simulink model "quadcopter_model"  (R2020b)
settings: Solver=VariableStepAuto  StartTime=0.0  StopTime=40  MaxStep=1e-3  RelTol=1e-3
values from neighbouring files (symbols this model uses):
  g = 9.81    [model_parameters.m]    (also in state_fcn.m = [0; 0; 9.81]; state_fcn1.m = [0; 0; 9.81])
  J = diag([Jxx, Jyy, Jzz])    [model_parameters.m]    (also in state_fcn1.m)
  JR = 1e-5    (= 1e-05)    [model_parameters.m]    (also in state_fcn1.m)
  Kv = 980    [model_parameters.m]
  m = 0.6    [model_parameters.m]    (also in state_fcn1.m)
  Omega_b = 0    [model_parameters.m]
  S = [cT cT cT cT ... (first row only)    [model_parameters.m]    (also in state_fcn1.m = [       cT              cT              cT              cT)
  Tm = 0.02    [model_parameters.m]
  Ts = 0.1    [linear_mpc.m]
  Ub = 12    [model_parameters.m]
libraries: simulink x5, eeStairGenerator x4, sharedutil x3, mpclib x1, robotcorelib x1
settings Model: Creator=Bojan  LastModifiedBy=Bojan Derajic

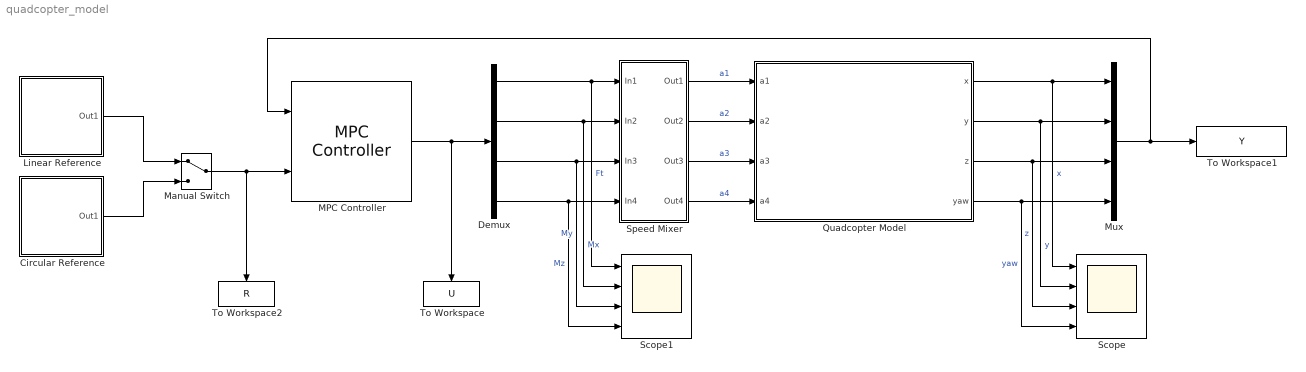
== system quadcopter_model ==
  Circular Reference : Subsystem
  Demux : Demux
  Linear Reference : Subsystem
  MPC Controller : mpclib/MPC Controller  SCDEnableBlockLinearizationSpecification=on  mpcobj=MPC_lin  is_multiple=0  enable_value=0  return_u0=off  updateMPCinCallerWorkspace=on  md_inport=off  mv_inport=off  uref_inport=off  return_cost=off  return_mvseq=off  return_qpstatus=off  return_xseq=off  return_state=off  return_ovseq=off  state_inport=off  umin_inport=off  umax_inport=off  ymin_inport=off  ymax_inport=off  cc_inport=off  ywt_inport=off  uwt_inport=off  duwt_inport=off  rhoeps_inport=off  pm_inport=off  MaximumP=10  HorizonChoice=FixedHorizon  n_ts=0.1  n_p=60  n_mv=4  n_md=0  n_ud=0  n_mo=4  n_uo=0  BlockDataType=double  SampleTimeInherited=off  switch_inport=off
  Manual Switch : ManualSwitch
  Mux : Mux
  Quadcopter Model : Subsystem
      mask Display: image('C:\Users\Bojan Derajic\OneDrive\Master studije - Predmeti BG\Robotski sistemi (13M051RS)\Quadcopter model\icons\quadcopter.jpg'); % Use "Edit Image" on toolstrip to change.
  Scope : Scope  NumInputPorts=4
  Scope1 : Scope  NumInputPorts=4
  Speed Mixer : Subsystem
  To Workspace : ToWorkspace  VariableName=U  SaveFormat=Structure With Time  SampleTime=-1
  To Workspace1 : ToWorkspace  VariableName=Y  SaveFormat=Structure With Time  SampleTime=-1
  To Workspace2 : ToWorkspace  VariableName=R  SaveFormat=Structure With Time  SampleTime=-1
  wires:
  Speed Mixer/4(Out4) -> Quadcopter Model/4(a4)  "a4"
  Speed Mixer/3(Out3) -> Quadcopter Model/3(a3)  "a3"
  Speed Mixer/2(Out2) -> Quadcopter Model/2(a2)  "a2"
  Speed Mixer/1(Out1) -> Quadcopter Model/1(a1)  "a1"
  Quadcopter Model/1(x) -> Scope/1, Mux/1  "x"
  Quadcopter Model/2(y) -> Mux/2, Scope/2  "y"
  Quadcopter Model/3(z) -> Mux/3, Scope/3  "z"
  Quadcopter Model/4(yaw) -> Mux/4, Scope/4  "yaw"
  Mux/1 -> To Workspace1/1, MPC Controller/1
  Demux/1 -> Scope1/1, Speed Mixer/1(In1)  "Ft"
  Demux/2 -> Scope1/2, Speed Mixer/2(In2)  "Mx"
  Demux/3 -> Scope1/3, Speed Mixer/3(In3)  "My"
  Demux/4 -> Scope1/4, Speed Mixer/4(In4)  "Mz"
  MPC Controller/1 -> To Workspace/1, Demux/1
  Manual Switch/1 -> MPC Controller/2, To Workspace2/1
  Linear Reference/1(Out1) -> Manual Switch/1
  Circular Reference/1(Out1) -> Manual Switch/2

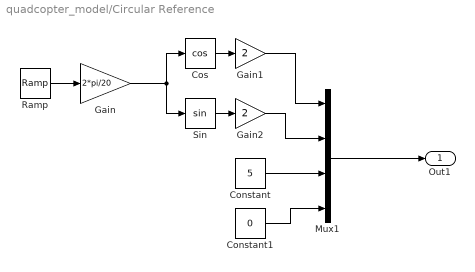
== system quadcopter_model/Circular Reference ==
  Constant : Constant  Value=5
  Constant1 : Constant  Value=0
  Cos : Trigonometry  Operator=cos
  Gain : Gain  Gain=2*pi/20
  Gain1 : Gain  Gain=2
  Gain2 : Gain  Gain=2
  Mux1 : Mux
  Ramp : simulink/Sources/Ramp  slope=1  start=5  InitialOutput=0
  Sin : Trigonometry
  Out1 : Outport
  wires:
  Gain1/1 -> Mux1/1
  Gain2/1 -> Mux1/2
  Cos/1 -> Gain1/1
  Sin/1 -> Gain2/1
  Ramp/1 -> Gain/1
  Mux1/1 -> Out1/1
  Constant/1 -> Mux1/3
  Gain/1 -> Sin/1, Cos/1
  Constant1/1 -> Mux1/4

== system quadcopter_model/Linear Reference ==
  Mux1 : Mux
  Stair Generator : eeStairGenerator/Stair Generator  LabelModeActiveChoice=Discrete  TimeInput=[5, 15]  AmplitudeInput=[-2, 3]  SampleTime=Ts  RepeatPattern=off  OutDataTypeStr=double
      settings: SourceProductBaseCode=PS
  Stair Generator1 : eeStairGenerator/Stair Generator  LabelModeActiveChoice=Discrete  TimeInput=[0, 24]  AmplitudeInput=[5, 0]  SampleTime=Ts  RepeatPattern=off  OutDataTypeStr=double
      settings: SourceProductBaseCode=PS
  Stair Generator2 : eeStairGenerator/Stair Generator  LabelModeActiveChoice=Discrete  TimeInput=[20]  AmplitudeInput=[0.1]  SampleTime=Ts  RepeatPattern=off  OutDataTypeStr=double
      settings: SourceProductBaseCode=PS
  Stair Generator3 : eeStairGenerator/Stair Generator  LabelModeActiveChoice=Discrete  TimeInput=[10]  AmplitudeInput=[5]  SampleTime=Ts  RepeatPattern=off  OutDataTypeStr=double
      settings: SourceProductBaseCode=PS
  Out1 : Outport
  wires:
  Stair Generator1/1 -> Mux1/3
  Stair Generator/1 -> Mux1/2
  Stair Generator2/1 -> Mux1/4
  Mux1/1 -> Out1/1
  Stair Generator3/1 -> Mux1/1

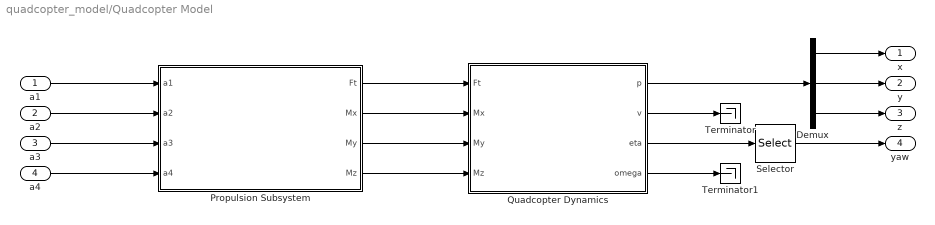
== system quadcopter_model/Quadcopter Model ==
  a1 : Inport
  a2 : Inport  Port=2
  a3 : Inport  Port=3
  a4 : Inport  Port=4
  Demux : Demux  Outputs=3
  Propulsion Subsystem : Subsystem
  Quadcopter Dynamics : Subsystem
  Selector : Selector  InputPortWidth=3  IndexOptions=Index vector (dialog)  Indices=[3]  OutputSizes=1
  Terminator : Terminator
  Terminator1 : Terminator
  x : Outport
  y : Outport  Port=2
  z : Outport  Port=3
  yaw : Outport  Port=4
  wires:
  Propulsion Subsystem/1(Ft) -> Quadcopter Dynamics/1(Ft)
  a4/1 -> Propulsion Subsystem/4(a4)
  a1/1 -> Propulsion Subsystem/1(a1)
  Propulsion Subsystem/3(My) -> Quadcopter Dynamics/3(My)
  a2/1 -> Propulsion Subsystem/2(a2)
  Propulsion Subsystem/2(Mx) -> Quadcopter Dynamics/2(Mx)
  Propulsion Subsystem/4(Mz) -> Quadcopter Dynamics/4(Mz)
  Quadcopter Dynamics/1(p) -> Demux/1
  a3/1 -> Propulsion Subsystem/3(a3)
  Quadcopter Dynamics/2(v) -> Terminator/1
  Quadcopter Dynamics/3(eta) -> Selector/1
  Quadcopter Dynamics/4(omega) -> Terminator1/1
  Demux/1 -> x/1
  Demux/2 -> y/1
  Demux/3 -> z/1
  Selector/1 -> yaw/1

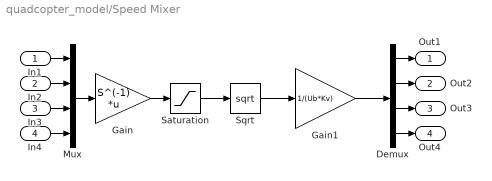
== system quadcopter_model/Speed Mixer ==
  In1 : Inport
  In2 : Inport  Port=2
  In3 : Inport  Port=3
  In4 : Inport  Port=4
  Demux : Demux
  Gain : Gain  Gain=S^(-1)  Multiplication=Matrix(K*u)
  Gain1 : Gain  Gain=1/(Ub*Kv)
  Mux : Mux
  Saturation : Saturate  UpperLimit=Inf  LowerLimit=0
  Sqrt : Sqrt  SaturateOnIntegerOverflow=on
  Out1 : Outport
  Out2 : Outport  Port=2
  Out3 : Outport  Port=3
  Out4 : Outport  Port=4
  wires:
  Demux/4 -> Out4/1
  Mux/1 -> Gain/1
  In1/1 -> Mux/1
  Gain1/1 -> Demux/1
  Demux/2 -> Out2/1
  Sqrt/1 -> Gain1/1
  In2/1 -> Mux/2
  Demux/1 -> Out1/1
  In4/1 -> Mux/4
  In3/1 -> Mux/3
  Demux/3 -> Out3/1
  Gain/1 -> Saturation/1
  Saturation/1 -> Sqrt/1

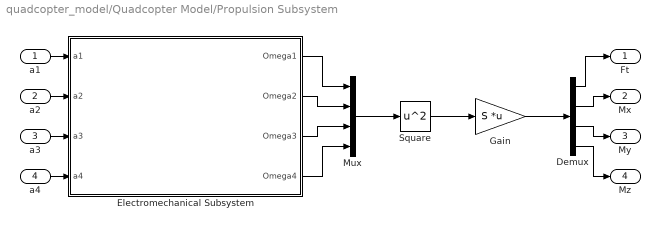
== system quadcopter_model/Quadcopter Model/Propulsion Subsystem ==
  a1 : Inport
  a2 : Inport  Port=2
  a3 : Inport  Port=3
  a4 : Inport  Port=4
  Demux : Demux
  Electromechanical Subsystem : Subsystem
  Gain : Gain  Gain=S  Multiplication=Matrix(K*u)
  Mux : Mux
  Square : Math  Operator=square  SaturateOnIntegerOverflow=on
  Ft : Outport
  Mx : Outport  Port=2
  My : Outport  Port=3
  Mz : Outport  Port=4
  wires:
  Electromechanical Subsystem/4(Omega4) -> Mux/4
  Electromechanical Subsystem/3(Omega3) -> Mux/3
  a1/1 -> Electromechanical Subsystem/1(a1)
  a4/1 -> Electromechanical Subsystem/4(a4)
  Gain/1 -> Demux/1
  Square/1 -> Gain/1
  a3/1 -> Electromechanical Subsystem/3(a3)
  Mux/1 -> Square/1
  Electromechanical Subsystem/1(Omega1) -> Mux/1
  Electromechanical Subsystem/2(Omega2) -> Mux/2
  a2/1 -> Electromechanical Subsystem/2(a2)
  Demux/1 -> Ft/1
  Demux/3 -> My/1
  Demux/2 -> Mx/1
  Demux/4 -> Mz/1

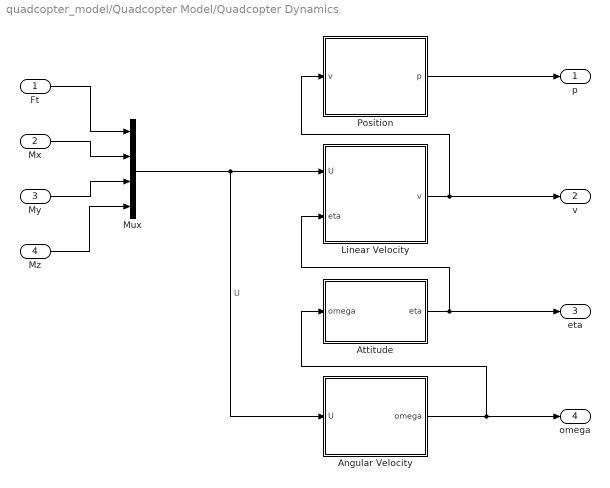
== system quadcopter_model/Quadcopter Model/Quadcopter Dynamics ==
  Ft : Inport
  Mx : Inport  Port=2
  My : Inport  Port=3
  Mz : Inport  Port=4
  Angular Velocity : Subsystem
  Attitude : Subsystem
  Linear Velocity : Subsystem
  Mux : Mux
  Position : Subsystem
  p : Outport
  v : Outport  Port=2
  eta : Outport  Port=3
  omega : Outport  Port=4
  wires:
  Mx/1 -> Mux/2
  Linear Velocity/1(v) -> Position/1(v), v/1
  Attitude/1(eta) -> eta/1, Linear Velocity/2(eta)
  Mux/1 -> Angular Velocity/1(U), Linear Velocity/1(U)  "U"
  Angular Velocity/1(omega) -> omega/1, Attitude/1(omega)
  Mz/1 -> Mux/4
  My/1 -> Mux/3
  Position/1(p) -> p/1
  Ft/1 -> Mux/1

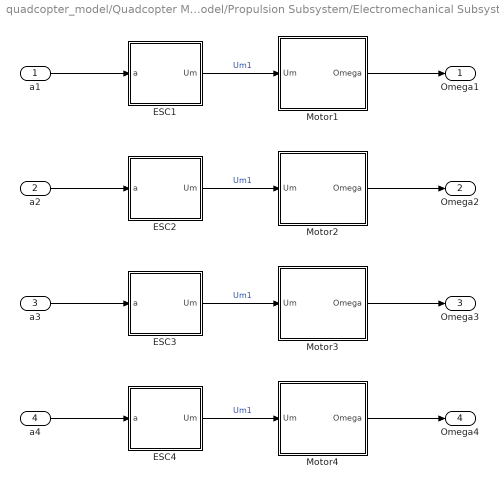
== system quadcopter_model/Quadcopter Model/Propulsion Subsystem/Electromechanical Subsystem ==
  a1 : Inport
  a2 : Inport  Port=2
  a3 : Inport  Port=3
  a4 : Inport  Port=4
  ESC1 : Subsystem
      mask Display: image('$imagefile'); % Use "Edit Image" on toolstrip to change.
  ESC2 : Subsystem
      mask Display: image('$imagefile'); % Use "Edit Image" on toolstrip to change.
  ESC3 : Subsystem
      mask Display: image('$imagefile'); % Use "Edit Image" on toolstrip to change.
  ESC4 : Subsystem
      mask Display: image('$imagefile'); % Use "Edit Image" on toolstrip to change.
  Motor1 : Subsystem
      mask Display: image('C:\Users\Bojan Derajic\OneDrive\Master studije - Predmeti BG\Robotski sistemi (13M051RS)\Quadcopter model\icons\motor.png'); % Use "Edit Image" on toolstrip to change.
  Motor2 : Subsystem
      mask Display: image('C:\Users\Bojan Derajic\OneDrive\Master studije - Predmeti BG\Robotski sistemi (13M051RS)\Quadcopter model\icons\motor.png'); % Use "Edit Image" on toolstrip to change.
  Motor3 : Subsystem
      mask Display: image('C:\Users\Bojan Derajic\OneDrive\Master studije - Predmeti BG\Robotski sistemi (13M051RS)\Quadcopter model\icons\motor.png'); % Use "Edit Image" on toolstrip to change.
  Motor4 : Subsystem
      mask Display: image('C:\Users\Bojan Derajic\OneDrive\Master studije - Predmeti BG\Robotski sistemi (13M051RS)\Quadcopter model\icons\motor.png'); % Use "Edit Image" on toolstrip to change.
  Omega1 : Outport
  Omega2 : Outport  Port=2
  Omega3 : Outport  Port=3
  Omega4 : Outport  Port=4
  wires:
  ESC1/1(Um) -> Motor1/1(Um)  "Um1"
  Motor1/1(Omega) -> Omega1/1
  a1/1 -> ESC1/1(a)
  a2/1 -> ESC2/1(a)
  ESC2/1(Um) -> Motor2/1(Um)  "Um1"
  Motor2/1(Omega) -> Omega2/1
  a3/1 -> ESC3/1(a)
  ESC3/1(Um) -> Motor3/1(Um)  "Um1"
  Motor3/1(Omega) -> Omega3/1
  a4/1 -> ESC4/1(a)
  ESC4/1(Um) -> Motor4/1(Um)  "Um1"
  Motor4/1(Omega) -> Omega4/1

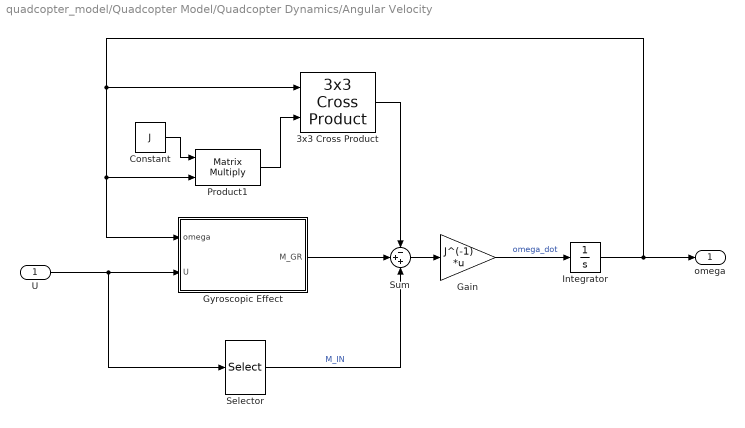
== system quadcopter_model/Quadcopter Model/Quadcopter Dynamics/Angular Velocity ==
  U : Inport
  3x3 Cross Product : sharedutil/3x3 Cross Product  aMode=aMode
      settings: SourceProductBaseCode=AE,PW,MT,UV,VE,VP
  Constant : Constant  Value=J
  Gain : Gain  Gain=J^(-1)  Multiplication=Matrix(K*u)
  Gyroscopic Effect : Subsystem
  Integrator : Integrator
  Product1 : Product  Multiplication=Matrix(*)
  Selector : Selector  InputPortWidth=4  IndexOptions=Index vector (dialog)  Indices=[2 3 4]  OutputSizes=1
  Sum : Sum  Inputs=-++
  omega : Outport
  wires:
  Constant/1 -> Product1/1
  U/1 -> Selector/1, Gyroscopic Effect/2(U)
  Integrator/1 -> omega/1, Gyroscopic Effect/1(omega), Product1/2, 3x3 Cross Product/1
  Sum/1 -> Gain/1
  3x3 Cross Product/1 -> Sum/1
  Product1/1 -> 3x3 Cross Product/2
  Gain/1 -> Integrator/1  "omega_dot"
  Selector/1 -> Sum/3  "M_IN"
  Gyroscopic Effect/1(M_GR) -> Sum/2

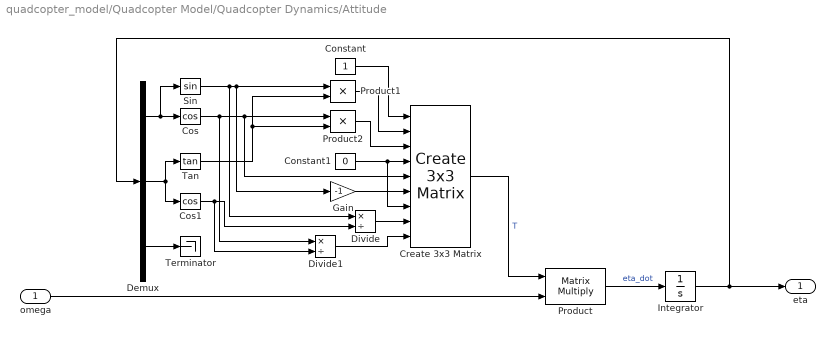
== system quadcopter_model/Quadcopter Model/Quadcopter Dynamics/Attitude ==
  omega : Inport
  Constant : Constant
  Constant1 : Constant  Value=0
  Cos : Trigonometry  Operator=cos
  Cos1 : Trigonometry  Operator=cos
  Create 3x3 Matrix : sharedutil/Create 3x3 Matrix  aMode=aMode
      settings: SourceProductBaseCode=AE,PW,MT,UV,VE,VP
  Demux : Demux  Outputs=3
  Divide : Product  Inputs=*/
  Divide1 : Product  Inputs=*/
  Gain : Gain  Gain=-1
  Integrator : Integrator
  Product : Product  Multiplication=Matrix(*)
  Product1 : Product
  Product2 : Product
  Sin : Trigonometry
  Tan : Trigonometry  Operator=tan
  Terminator : Terminator
  eta : Outport
  wires:
  Integrator/1 -> Demux/1, eta/1
  omega/1 -> Product/2
  Product/1 -> Integrator/1  "eta_dot"
  Create 3x3 Matrix/1 -> Product/1  "T"
  Demux/3 -> Terminator/1
  Constant/1 -> Create 3x3 Matrix/1
  Constant1/1 -> Create 3x3 Matrix/4, Create 3x3 Matrix/7
  Demux/1 -> Sin/1, Cos/1
  Demux/2 -> Cos1/1, Tan/1
  Product1/1 -> Create 3x3 Matrix/2
  Tan/1 -> Product2/2, Product1/2
  Sin/1 -> Divide/1, Gain/1, Product1/1
  Product2/1 -> Create 3x3 Matrix/3
  Cos/1 -> Divide1/1, Create 3x3 Matrix/5, Product2/1
  Gain/1 -> Create 3x3 Matrix/6
  Divide/1 -> Create 3x3 Matrix/8
  Divide1/1 -> Create 3x3 Matrix/9
  Cos1/1 -> Divide1/2, Divide/2

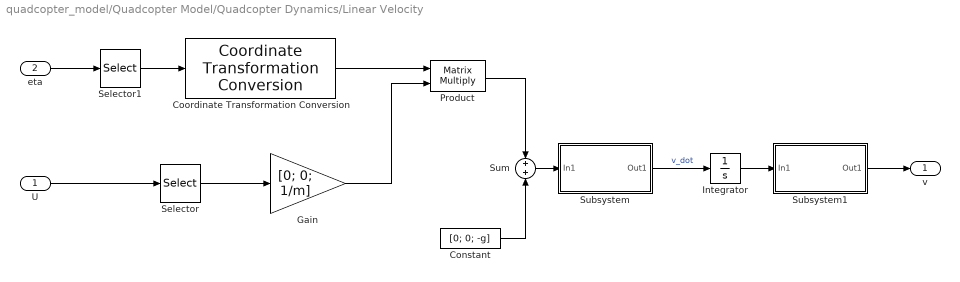
== system quadcopter_model/Quadcopter Model/Quadcopter Dynamics/Linear Velocity ==
  U : Inport
  eta : Inport  Port=2
  Constant : Constant  Value=[0; 0; -g]
  Coordinate Transformation Conversion : robotcorelib/Coordinate Transformation Conversion  InputRepresentation=Euler Angles  InputEulerSequence=ZYX  ShowTrVecInputPort=on  OutputRepresentation=Rotation Matrix  OutputEulerSequence=ZYX  ShowTrVecOutputPort=on  SimulateUsing=Interpreted execution
      settings: SourceProductBaseCode=NV,RO,RR,UV
  Gain : Gain  Gain=[0; 0; 1/m]
  Integrator : Integrator
  Product : Product  Multiplication=Matrix(*)
  Selector : Selector  InputPortWidth=4  IndexOptions=Index vector (dialog)  Indices=[1]  OutputSizes=1
  Selector1 : Selector  InputPortWidth=3  IndexOptions=Index vector (dialog)  Indices=[3 2 1]  OutputSizes=1
  Subsystem : Subsystem
  Subsystem1 : Subsystem
  Sum : Sum
  v : Outport
  wires:
  Integrator/1 -> Subsystem1/1(In1)
  Coordinate Transformation Conversion/1 -> Product/1
  Selector/1 -> Gain/1
  U/1 -> Selector/1
  Subsystem1/1(Out1) -> v/1
  Subsystem/1(Out1) -> Integrator/1  "v_dot"
  Sum/1 -> Subsystem/1(In1)
  Gain/1 -> Product/2
  Constant/1 -> Sum/2
  Product/1 -> Sum/1
  Selector1/1 -> Coordinate Transformation Conversion/1
  eta/1 -> Selector1/1

== system quadcopter_model/Quadcopter Model/Quadcopter Dynamics/Position ==
  v : Inport
  Integrator : Integrator
  Selector : Selector  InputPortWidth=3  IndexOptions=Index vector (dialog)  Indices=[3]  OutputSizes=1
  p : Outport
  tag scope: z=global
  wires:
  v/1 -> Integrator/1  "p_dot"
  Integrator/1 -> Selector/1, p/1
  Selector/1 -> [z]

== system quadcopter_model/Quadcopter Model/Propulsion Subsystem/Electromechanical Subsystem/ESC1 ==
  a : Inport
  Constant : Constant  Value=Ub
  Product : Product
  Um : Outport
  wires:
  a/1 -> Product/1
  Constant/1 -> Product/2
  Product/1 -> Um/1

== system quadcopter_model/Quadcopter Model/Propulsion Subsystem/Electromechanical Subsystem/ESC2 ==
  a : Inport
  Constant : Constant  Value=Ub
  Product : Product
  Um : Outport
  wires:
  Product/1 -> Um/1
  Constant/1 -> Product/2
  a/1 -> Product/1

== system quadcopter_model/Quadcopter Model/Propulsion Subsystem/Electromechanical Subsystem/ESC3 ==
  a : Inport
  Constant : Constant  Value=Ub
  Product : Product
  Um : Outport
  wires:
  a/1 -> Product/1
  Constant/1 -> Product/2
  Product/1 -> Um/1

== system quadcopter_model/Quadcopter Model/Propulsion Subsystem/Electromechanical Subsystem/ESC4 ==
  a : Inport
  Constant : Constant  Value=Ub
  Product : Product
  Um : Outport
  wires:
  Product/1 -> Um/1
  Constant/1 -> Product/2
  a/1 -> Product/1

== system quadcopter_model/Quadcopter Model/Propulsion Subsystem/Electromechanical Subsystem/Motor1 ==
  Um : Inport
  Constant : Constant  Value=Kv
  Constant1 : Constant  Value=Omega_b
  Product : Product
  Sum : Sum  Inputs=|++
  Transfer Fcn : TransferFcn  Denominator=[Tm 1]
  Omega : Outport
  wires:
  Um/1 -> Product/1
  Sum/1 -> Transfer Fcn/1
  Constant/1 -> Product/2
  Product/1 -> Sum/1
  Constant1/1 -> Sum/2
  Transfer Fcn/1 -> Omega/1

== system quadcopter_model/Quadcopter Model/Propulsion Subsystem/Electromechanical Subsystem/Motor2 ==
  Um : Inport
  Constant : Constant  Value=Kv
  Constant1 : Constant  Value=Omega_b
  Product : Product
  Sum : Sum  Inputs=|++
  Transfer Fcn : TransferFcn  Denominator=[Tm 1]
  Omega : Outport
  wires:
  Transfer Fcn/1 -> Omega/1
  Constant1/1 -> Sum/2
  Product/1 -> Sum/1
  Constant/1 -> Product/2
  Sum/1 -> Transfer Fcn/1
  Um/1 -> Product/1

== system quadcopter_model/Quadcopter Model/Propulsion Subsystem/Electromechanical Subsystem/Motor3 ==
  Um : Inport
  Constant : Constant  Value=Kv
  Constant1 : Constant  Value=Omega_b
  Product : Product
  Sum : Sum  Inputs=|++
  Transfer Fcn : TransferFcn  Denominator=[Tm 1]
  Omega : Outport
  wires:
  Um/1 -> Product/1
  Sum/1 -> Transfer Fcn/1
  Constant/1 -> Product/2
  Product/1 -> Sum/1
  Constant1/1 -> Sum/2
  Transfer Fcn/1 -> Omega/1

== system quadcopter_model/Quadcopter Model/Propulsion Subsystem/Electromechanical Subsystem/Motor4 ==
  Um : Inport
  Constant : Constant  Value=Kv
  Constant1 : Constant  Value=Omega_b
  Product : Product
  Sum : Sum  Inputs=|++
  Transfer Fcn : TransferFcn  Denominator=[Tm 1]
  Omega : Outport
  wires:
  Transfer Fcn/1 -> Omega/1
  Constant1/1 -> Sum/2
  Product/1 -> Sum/1
  Constant/1 -> Product/2
  Sum/1 -> Transfer Fcn/1
  Um/1 -> Product/1

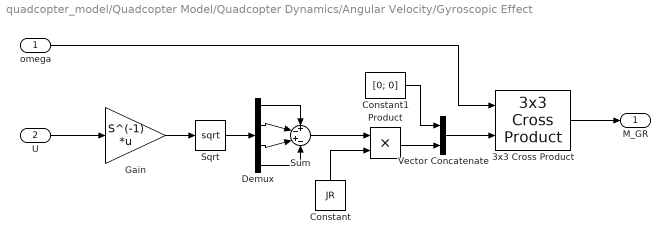
== system quadcopter_model/Quadcopter Model/Quadcopter Dynamics/Angular Velocity/Gyroscopic Effect ==
  omega : Inport
  U : Inport  Port=2
  3x3 Cross Product : sharedutil/3x3 Cross Product  aMode=aMode
      settings: SourceProductBaseCode=AE,PW,MT,UV,VE,VP
  Constant : Constant  Value=JR
  Constant1 : Constant  Value=[0; 0]
  Demux : Demux
  Gain : Gain  Gain=S^(-1)  Multiplication=Matrix(K*u)
  Product : Product
  Sqrt : Sqrt  SaturateOnIntegerOverflow=on
  Sum : Sum  Inputs=+-+-
  Vector Concatenate : Concatenate
  M_GR : Outport
  wires:
  Constant/1 -> Product/2
  Demux/3 -> Sum/3
  Demux/4 -> Sum/4
  Constant1/1 -> Vector Concatenate/1
  Sqrt/1 -> Demux/1
  Demux/1 -> Sum/1
  Gain/1 -> Sqrt/1
  Demux/2 -> Sum/2
  Sum/1 -> Product/1
  Product/1 -> Vector Concatenate/2
  U/1 -> Gain/1
  3x3 Cross Product/1 -> M_GR/1
  Vector Concatenate/1 -> 3x3 Cross Product/2
  omega/1 -> 3x3 Cross Product/1

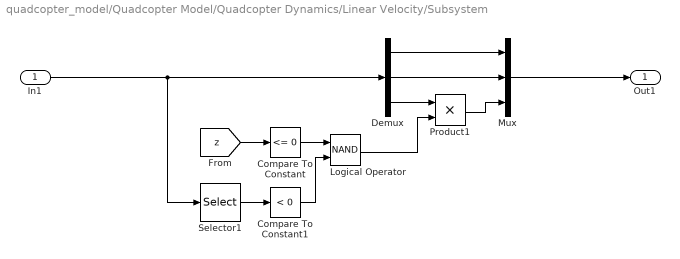
== system quadcopter_model/Quadcopter Model/Quadcopter Dynamics/Linear Velocity/Subsystem ==
  In1 : Inport
  Compare To Constant : simulink/Logic and Bit Operations/Compare To Constant  relop=<=  const=0  OutDataTypeStr=boolean
  Compare To Constant1 : simulink/Logic and Bit Operations/Compare To Constant  relop=<  const=0  OutDataTypeStr=boolean  ZeroCross=off
  Demux : Demux  Outputs=3
  Logical Operator : Logic  Operator=NAND  AllPortsSameDT=off  OutDataTypeStr=boolean
  Mux : Mux  Inputs=3
  Product1 : Product
  Selector1 : Selector  InputPortWidth=3  IndexOptions=Index vector (dialog)  Indices=[3]  OutputSizes=1
  Out1 : Outport
  wires:
  Demux/1 -> Mux/1
  [z] -> Compare To Constant/1
  Logical Operator/1 -> Product1/2
  Selector1/1 -> Compare To Constant1/1
  Compare To Constant1/1 -> Logical Operator/2
  In1/1 -> Selector1/1, Demux/1
  Compare To Constant/1 -> Logical Operator/1
  Demux/2 -> Mux/2
  Product1/1 -> Mux/3
  Demux/3 -> Product1/1
  Mux/1 -> Out1/1

== system quadcopter_model/Quadcopter Model/Quadcopter Dynamics/Linear Velocity/Subsystem1 ==
  In1 : Inport
  Compare To Constant : simulink/Logic and Bit Operations/Compare To Constant  relop=<=  const=0  OutDataTypeStr=boolean
  Compare To Constant1 : simulink/Logic and Bit Operations/Compare To Constant  relop=<  const=0  OutDataTypeStr=boolean  ZeroCross=off
  Demux : Demux  Outputs=3
  Logical Operator : Logic  Operator=NAND  AllPortsSameDT=off  OutDataTypeStr=boolean
  Mux : Mux  Inputs=3
  Product1 : Product
  Selector1 : Selector  InputPortWidth=3  IndexOptions=Index vector (dialog)  Indices=[3]  OutputSizes=1
  Out1 : Outport
  wires:
  Demux/3 -> Product1/1
  Product1/1 -> Mux/3
  Demux/2 -> Mux/2
  Compare To Constant/1 -> Logical Operator/1
  In1/1 -> Demux/1, Selector1/1
  Compare To Constant1/1 -> Logical Operator/2
  Selector1/1 -> Compare To Constant1/1
  Logical Operator/1 -> Product1/2
  [z] -> Compare To Constant/1
  Demux/1 -> Mux/1
  Mux/1 -> Out1/1
